simulink model "ROB_512_HW6_Hybrid"  (R2015a)
settings: Solver=ode23t  StartTime=0.0  StopTime=1.5  MaxStep=0.001  RelTol=1e-3
InitFcn:
  | Ka = 2;
  | Kb = 50;
libraries: fl_lib x17, nesl_utility x8, sh_lib x6, vrlib x3, simulink x2
Description:
  | Closed-Loop Electrohydraulic Actuator with Proportional Valve
  | 
  | This example shows an actuator that consists of a proportional 4-way directional valve
  | driving a double-acting hydraulic cylinder. The cylinder drives a load consisting of a mass,
  | viscous and Coulomb friction, constant force, and a spring. The actuator is powered
  | by a variable-displacement, pressure-compensated pump, driven by a constant velocity
  | motor. Pipelines between the valve, cylinder, pump, and the tank are simulated
  | with the Hydraulic Pipeline blocks.
  | 
  | 
  | Copyright 2008-2015 The MathWorks, Inc.
settings Model: ExtModeAutoUpdateStatusClock=off  Creator=MathWorks  LastModifiedBy=Ramsey
settings DataIOCC: SignalLoggingSaveFormat=ModelDataLogs
settings OptimizationCC: ExpressionDepthLimit=2147483647  InitFltsAndDblsToZero=on
settings DebuggingCC: SaveWithParameterizedLinksMsg=none  UnderspecifiedInitializationDetection=Classic  MergeDetectMultiDrivingBlocksExec=none  SignalResolutionControl=TryResolveAllWithWarning  SolverPrmCheckMsg=warning  MultiTaskDSMMsg=warning  FcnCallInpInsideContextMsg=UseLocalSettings  StateNameClashWarn=warning
settings GRTTargetCC: TargetFcnLib=ansi_tfl_tmw.mat  CombineOutputUpdateFcns=off  GRTInterface=on

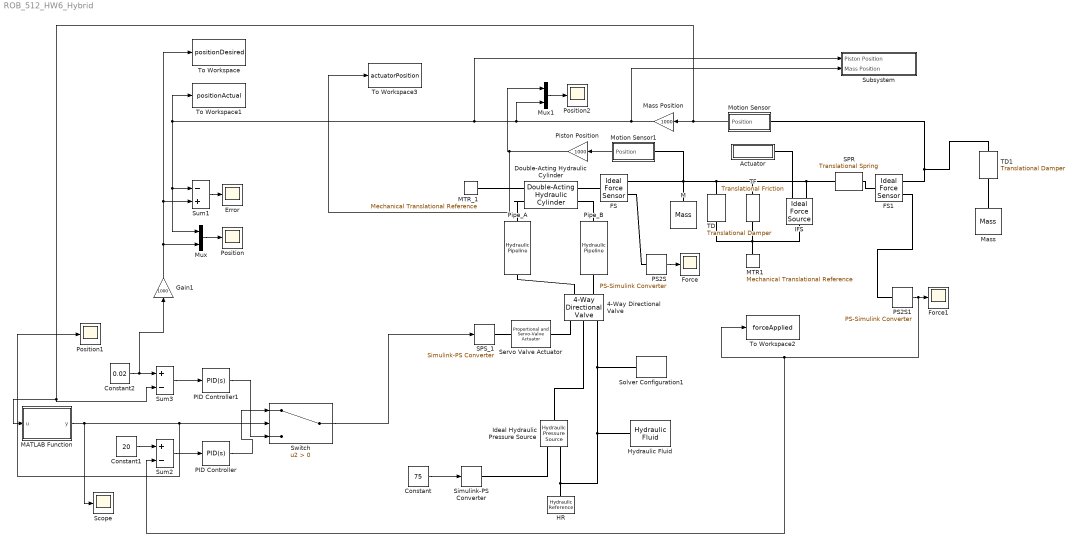
== system ROB_512_HW6_Hybrid ==
  4-Way Directional Valve : sh_lib/Valves/Directional Valves/4-Way Directional Valve  Tag=Factory Generic  mdl_type=1  area_max=0.00015 m^2  opening_max=0.01 m  opening_tab=[-0.002 0 0.005 0.015] m  area_tab=[1e-12 4e-12 1e-05 1.02e-05] m^2  pressure_tab=[-5000000 -2000000 2000000 5000000] Pa  flow_rate_tab=[-1e-12 -6e-14 6000000000000 100000000000;-8e-08 -4e-08 4000000 8000000;-0.0025 -0.00103 0.001 0.0024;-0.00258 -0.001032 0.00106 0.00247] m^3/s  interp_method=1  extrap_method=1  C_d=0.7  x_0_P_A=1e-05 m  x_0_P_B=1e-05 m  x_0_A_T=1e-05 m  x_0_B_T=1e-05 m  Re_cr=12  A_leak=1e-12 m^2
  Actuator : Subsystem
  Constant : Constant  Value=75
  Constant1 : Constant  Value=20
  Constant2 : Constant  Value=0.02
  Double-Acting Hydraulic Cylinder : sh_lib/Hydraulic Cylinders/Double-Acting Hydraulic Cylinder  Tag=Factory Generic  area_A=0.004 m^2  area_B=0.002 m^2  stroke=0.2 m  init_pos=0.1 m  dead_vol_A=0.001 m^3  dead_vol_B=0.001 m^3  init_pressure_A=0 Pa  init_pressure_B=0 Pa  k_sh=1.4  stiff=1e+12 N/m  D=150 N/(m/s)  or=1  or_sign=1
  Error : Scope
      settings: TimeRange=10  YMin=-0.01  YMax=0.02  MaxDataPoints=500000
  FS : fl_lib/Mechanical/Mechanical Sensors/Ideal Force Sensor  Tag=Factory Generic
  FS1 : fl_lib/Mechanical/Mechanical Sensors/Ideal Force Sensor  Tag=Factory Generic
  Force : Scope
      settings: TimeRange=3  YMin=-17500  YMax=27500  MaxDataPoints=500000
  Force1 : Scope
      settings: TimeRange=1.5  YMin=0  YMax=100  SaveName=ScopeData3  MaxDataPoints=500000
  Gain1 : Gain  Gain=1000
  HR : fl_lib/Hydraulic/Hydraulic Elements/Hydraulic Reference  Tag=Factory Generic
  Hydraulic Fluid : sh_lib/Hydraulic Utilities/Hydraulic Fluid  Tag=Factory Generic  DataSource=1  SelFluid=7  SysTemp=60 c  TrapAir=0.005  ViscDerFactor=1  range_error=2
  IFS : fl_lib/Mechanical/Mechanical Sources/Ideal Force Source  Tag=Factory Generic
  Ideal Hydraulic Pressure Source : fl_lib/Hydraulic/Hydraulic Sources/Hydraulic Pressure Source  Tag=Factory Generic
  M : fl_lib/Mechanical/Translational Elements/Mass  Tag=Factory Generic  mass=10 kg  v_specify=on  v_priority=High  v=0 m/s  f_specify=off  f_priority=High  f=0 N
  MATLAB Function : MATLAB Function  TreatAsAtomicUnit=on
  MTR1 : fl_lib/Mechanical/Translational Elements/Mechanical Translational Reference  Tag=Factory Generic
  MTR_1 : fl_lib/Mechanical/Translational Elements/Mechanical Translational Reference  Tag=Factory Generic
  Mass : fl_lib/Mechanical/Translational Elements/Mass  mass=5000 kg  v_specify=off  v_priority=High  v=0 m/s  f_specify=off  f_priority=High  f=0 N
  Mass Position : Gain  Gain=1000
  Motion Sensor : Subsystem
  Motion Sensor1 : Subsystem
  Mux : Mux  Inputs=2
  Mux1 : Mux  Inputs=2
  PID Controller : simulink/Continuous/PID Controller  Controller=PID  TimeDomain=Continuous-time  SampleTime=-1  IntegratorMethod=Forward Euler  FilterMethod=Forward Euler  Form=Parallel  UseFilter=on  ControllerParametersSource=internal  P=0.00035  I=0.00005  D=0  N=100  InitialConditionSource=internal  InitialConditionForIntegrator=0  InitialConditionForFilter=0  ExternalReset=none  LimitOutput=off  UpperSaturationLimit=inf  LowerSaturationLimit=-inf  LinearizeAsGain=on  AntiWindupMode=none  Kb=1  TrackingMode=off  Kt=1  PParamMin=[]  PParamMax=[]  IParamMin=[]  IParamMax=[]  DParamMin=[]  DParamMax=[]  NParamMin=[]  NParamMax=[]  KbParamMin=[]  KbParamMax=[]  KtParamMin=[]  KtParamMax=[]  POutMin=[]  POutMax=[]  IOutMin=[]  IOutMax=[]  DOutMin=[]  DOutMax=[]  NOutMin=[]  NOutMax=[]  KbOutMin=[]  KbOutMax=[]  KtOutMin=[]  KtOutMax=[]  IntegratorOutMin=[]  IntegratorOutMax=[]  FilterOutMin=[]  FilterOutMax=[]  SumOutMin=[]  SumOutMax=[]  SumI1OutMin=[]  SumI1OutMax=[]  SumI2OutMin=[]  SumI2OutMax=[]  SumI3OutMin=[]  SumI3OutMax=[]  SumDOutMin=[]  SumDOutMax=[]  SaturationOutMin=[]  SaturationOutMax=[]  IntegratorContinuousStateAttributes=''  IntegratorStateMustResolveToSignalObject=off  IntegratorRTWStateStorageClass=Auto  FilterContinuousStateAttributes=''  FilterStateMustResolveToSignalObject=off  FilterRTWStateStorageClass=Auto  DifferentiatorICPrevScaledInput=0  DifferentiatorOutMin=[]  DifferentiatorOutMax=[]
  PID Controller1 : simulink/Continuous/PID Controller  Controller=PID  TimeDomain=Continuous-time  SampleTime=-1  IntegratorMethod=Forward Euler  FilterMethod=Forward Euler  Form=Parallel  UseFilter=on  ControllerParametersSource=internal  P=5  I=0.1  D=0.2  N=100  InitialConditionSource=internal  InitialConditionForIntegrator=0  InitialConditionForFilter=0  ExternalReset=none  LimitOutput=off  UpperSaturationLimit=inf  LowerSaturationLimit=-inf  LinearizeAsGain=on  AntiWindupMode=none  Kb=1  TrackingMode=off  Kt=1  PParamMin=[]  PParamMax=[]  IParamMin=[]  IParamMax=[]  DParamMin=[]  DParamMax=[]  NParamMin=[]  NParamMax=[]  KbParamMin=[]  KbParamMax=[]  KtParamMin=[]  KtParamMax=[]  POutMin=[]  POutMax=[]  IOutMin=[]  IOutMax=[]  DOutMin=[]  DOutMax=[]  NOutMin=[]  NOutMax=[]  KbOutMin=[]  KbOutMax=[]  KtOutMin=[]  KtOutMax=[]  IntegratorOutMin=[]  IntegratorOutMax=[]  FilterOutMin=[]  FilterOutMax=[]  SumOutMin=[]  SumOutMax=[]  SumI1OutMin=[]  SumI1OutMax=[]  SumI2OutMin=[]  SumI2OutMax=[]  SumI3OutMin=[]  SumI3OutMax=[]  SumDOutMin=[]  SumDOutMax=[]  SaturationOutMin=[]  SaturationOutMax=[]  IntegratorContinuousStateAttributes=''  IntegratorStateMustResolveToSignalObject=off  IntegratorRTWStateStorageClass=Auto  FilterContinuousStateAttributes=''  FilterStateMustResolveToSignalObject=off  FilterRTWStateStorageClass=Auto  DifferentiatorICPrevScaledInput=0  DifferentiatorOutMin=[]  DifferentiatorOutMax=[]
  PS2S : nesl_utility/PS-Simulink Converter  PhysicalDomain=network_engine_domain  SubClassName=ps_output  LeftPortType=input  RightPortType=output  PseudoPeriodic=off  Frequencies=[]  Unit=1  AffineConversion=off
  PS2S1 : nesl_utility/PS-Simulink Converter  PhysicalDomain=network_engine_domain  SubClassName=ps_output  LeftPortType=input  RightPortType=output  PseudoPeriodic=off  Frequencies=[]  Unit=1  AffineConversion=off
  Pipe_A : sh_lib/Pipelines/Hydraulic Pipeline  Tag=Factory Generic  cs_type=1  d_in=0.02 m  area=0.0001 m^2  D_h=0.0112 m  s_factor=64  length=3 m  length_ad=2 m  roughness=1.5e-05 m  Re_lam=2000  Re_turb=4000  wall_type=1  pr_r_coef=2e-10 m/Pa  time_const=0.008 s  k_sh=1.4  initial_pressure=0 Pa
  Pipe_B : sh_lib/Pipelines/Hydraulic Pipeline  Tag=Factory Generic  cs_type=1  d_in=0.02 m  area=0.0001 m^2  D_h=0.0112 m  s_factor=64  length=3 m  length_ad=2 m  roughness=1.5e-05 m  Re_lam=2000  Re_turb=4000  wall_type=1  pr_r_coef=2e-10 m/Pa  time_const=0.008 s  k_sh=1.4  initial_pressure=0 Pa
  Piston Position : Gain  Gain=1000
  Position : Scope
      settings: TimeRange=1.5  YMin=2.5  YMax=20  SaveName=ScopeData2  MaxDataPoints=500000
  Position1 : Scope
      settings: TimeRange=3  YMin=1  YMax=1  SaveName=ScopeData5  MaxDataPoints=500000
  Position2 : Scope
      settings: ShowLegends=on  TimeRange=3  YMin=-10  YMax=150  SaveName=ScopeData6  MaxDataPoints=500000
  SPR : fl_lib/Mechanical/Translational Elements/Translational Spring  Tag=Factory Generic  spr_rate=1000 N/m  v_specify=off  v_priority=High  v=0 m/s  f_specify=off  f_priority=High  f=0 N  x_specify=on  x_priority=High  x=0 m
  SPS_1 : nesl_utility/Simulink-PS Converter  PhysicalDomain=network_engine_domain  SubClassName=ps_input  LeftPortType=input  RightPortType=output  PseudoPeriodic=off  Frequencies=[]  NoiseDistribution=none  NoiseParameters=[]  Unit=1  AffineConversion=off  InputFiltering=off  SimscapeFilterOrder=1  InputFilterTimeConstant=.001  UdotUserProvided=0
  Scope : Scope
      settings: SaveName=ScopeData4
  Servo Valve Actuator : sh_lib/Valves/Valve Actuators/Proportional and Servo-Valve Actuator  Tag=Factory Generic  gain=250  time_constant=0.002 s  saturation=0.3
  Simulink-PS Converter : nesl_utility/Simulink-PS Converter  PhysicalDomain=network_engine_domain  SubClassName=ps_input  LeftPortType=input  RightPortType=output  PseudoPeriodic=off  Frequencies=[]  NoiseDistribution=none  NoiseParameters=[]  Unit=bar  AffineConversion=off  InputFiltering=off  SimscapeFilterOrder=1  InputFilterTimeConstant=.001  UdotUserProvided=0
  Solver Configuration1 : nesl_utility/Solver Configuration  PhysicalDomain=network_engine_domain  SubClassName=solver  LeftPortType=input  RightPortType=generic  Accelerate=off  Tones=[]  Harmonics=[]  SimulateNoise=off  Profile=off  UseLocalSampling=off  EnableSwitchedLinearOptims=on  FrequencyDomain=off  UseCCode=off  RelTol=0.001  AbsTol=1e-06  MinStep=1e-09  ToWorkspace=off  RevertToSquareIcSolve=off  NumHomotopyIterations=100  DoDC=off  ResidualTolerance=1e-9  UseLocalSolver=off  LocalSolverChoice=NE_BACKWARD_EULER_ADVANCER  LocalSolverSampleTime=.001  DoFixedCost=off  MaxNonlinIter=3  MaxModeIter=2  LinearAlgebra=Sparse  DelaysMemoryBudget=1024  AutomaticFiltering=on  FilteringTimeConstant=0.001
  Subsystem : Subsystem
  Sum1 : Sum  Inputs=-+
  Sum2 : Sum  Inputs=+-
  Sum3 : Sum  Inputs=+-
  Switch : Switch  Criteria=u2 > Threshold  RndMeth=Round  ZeroCross=off
  TD : fl_lib/Mechanical/Translational Elements/Translational Damper  Tag=Factory Generic  D=2 N/(m/s)  v_specify=off  v_priority=High  v=0 m/s  f_specify=off  f_priority=High  f=0 N
  TD1 : fl_lib/Mechanical/Translational Elements/Translational Damper  Tag=Factory Generic  D=500 N/(m/s)  v_specify=off  v_priority=High  v=0 m/s  f_specify=off  f_priority=High  f=0 N
  TF : fl_lib/Mechanical/Translational Elements/Translational Friction  Tag=Factory Generic  brkwy_frc=500 N  Col_frc=500 N  visc_coef=0.01 N/(m/s)  trans_coef=10 s/m  vel_thr=0.0001 m/s  v_specify=off  v_priority=High  v=0 m/s  f_specify=off  f_priority=High  f=0 N
  To Workspace : ToWorkspace  VariableName=positionDesired  SaveFormat=Timeseries  SampleTime=-1
  To Workspace1 : ToWorkspace  VariableName=positionActual  SaveFormat=Timeseries  SampleTime=-1
  To Workspace2 : ToWorkspace  VariableName=forceApplied  SaveFormat=Timeseries  SampleTime=-1
  To Workspace3 : ToWorkspace  VariableName=actuatorPosition  SaveFormat=Timeseries  SampleTime=-1
  wires:
  PS2S/1 -> Force/1
  Constant1/1 -> Sum2/1
  Mux/1 -> Position/1
  Sum1/1 -> Error/1
  Constant/1 -> Simulink-PS Converter/1
  Gain1/1 -> To Workspace/1, Sum1/2, Mux/2
  PS2S1/1 -> To Workspace2/1, Sum2/2, Force1/1
  Sum2/1 -> PID Controller/1
  Constant2/1 -> Gain1/1, Sum3/1
  Sum3/1 -> PID Controller1/1
  Motion Sensor/1(Position) -> Mass Position/1, MATLAB Function/1(u), Sum3/2
  PID Controller/1 -> Switch/1
  PID Controller1/1 -> Switch/3
  Switch/1 -> SPS_1/1
  MATLAB Function/1(y) -> Scope/1, Position1/1, Switch/2
  Mux1/1 -> Position2/1
  Motion Sensor1/1(Position) -> Piston Position/1
  Piston Position/1 -> To Workspace3/1, Mux1/1
  Mass Position/1 -> Subsystem/2(Mass Position), Mux1/2, Subsystem/1(Piston Position), Mux/1, Sum1/1, To Workspace1/1
  connections:
  MTR_1/LConn1 -- Double-Acting Hydraulic Cylinder/LConn1
  FS/LConn1 -- Double-Acting Hydraulic Cylinder/RConn1
  FS/RConn2 -- PS2S/LConn1
  Ideal Hydraulic Pressure Source/RConn2 -- Hydraulic Fluid/RConn1 -- Solver Configuration1/RConn1 -- 4-Way Directional Valve/RConn3 -- HR/LConn1
  4-Way Directional Valve/RConn1 -- Servo Valve Actuator/RConn1
  SPS_1/RConn1 -- Servo Valve Actuator/LConn1
  Ideal Hydraulic Pressure Source/LConn1 -- 4-Way Directional Valve/RConn2
  SPR/LConn1 -- IFS/RConn2 -- TD/LConn1 -- Motion Sensor1/LConn1 -- M/LConn1 -- FS/RConn1 -- TF/LConn1
  Actuator/RConn1 -- IFS/RConn1
  TD/RConn1 -- TF/RConn1 -- IFS/LConn1 -- MTR1/LConn1
  Simulink-PS Converter/RConn1 -- Ideal Hydraulic Pressure Source/RConn1
  Double-Acting Hydraulic Cylinder/LConn2 -- Pipe_A/RConn1
  4-Way Directional Valve/LConn1 -- Pipe_A/LConn1
  Double-Acting Hydraulic Cylinder/RConn2 -- Pipe_B/LConn1
  4-Way Directional Valve/LConn2 -- Pipe_B/RConn1
  FS1/LConn1 -- SPR/RConn1
  Motion Sensor/LConn1 -- TD1/LConn1 -- FS1/RConn1
  FS1/RConn2 -- PS2S1/LConn1
  Mass/LConn1 -- TD1/RConn1

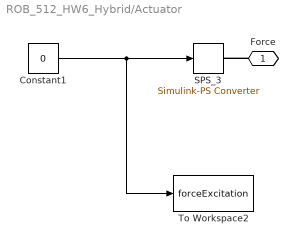
== system ROB_512_HW6_Hybrid/Actuator ==
  Constant1 : Constant  Value=0
  SPS_3 : nesl_utility/Simulink-PS Converter  PhysicalDomain=network_engine_domain  SubClassName=ps_input  LeftPortType=input  RightPortType=output  PseudoPeriodic=off  Frequencies=[]  NoiseDistribution=none  NoiseParameters=[]  Unit=1  AffineConversion=off  InputFiltering=off  SimscapeFilterOrder=1  InputFilterTimeConstant=.001  UdotUserProvided=0
  To Workspace2 : ToWorkspace  VariableName=forceExcitation  SaveFormat=Timeseries  SampleTime=-1
  Force : PMIOPort  Port=1  Side=Right
  wires:
  Constant1/1 -> To Workspace2/1, SPS_3/1
  connections:
  Force/RConn1 -- SPS_3/RConn1

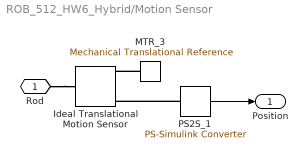
== system ROB_512_HW6_Hybrid/Motion Sensor ==
  Ideal Translational Motion Sensor : fl_lib/Mechanical/Mechanical Sensors/Ideal Translational Motion Sensor  Tag=Factory Generic  offset=0 m
  MTR_3 : fl_lib/Mechanical/Translational Elements/Mechanical Translational Reference  Tag=Factory Generic
  PS2S_1 : nesl_utility/PS-Simulink Converter  PhysicalDomain=network_engine_domain  SubClassName=ps_output  LeftPortType=input  RightPortType=output  PseudoPeriodic=off  Frequencies=[]  Unit=1  AffineConversion=off
  Rod : PMIOPort  Port=1  Side=Left
  Position : Outport
  wires:
  PS2S_1/1 -> Position/1
  connections:
  Rod/RConn1 -- Ideal Translational Motion Sensor/LConn1
  PS2S_1/LConn1 -- Ideal Translational Motion Sensor/RConn3
  MTR_3/LConn1 -- Ideal Translational Motion Sensor/RConn1

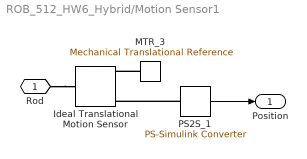
== system ROB_512_HW6_Hybrid/Motion Sensor1 ==
  Ideal Translational Motion Sensor : fl_lib/Mechanical/Mechanical Sensors/Ideal Translational Motion Sensor  Tag=Factory Generic  offset=0 m
  MTR_3 : fl_lib/Mechanical/Translational Elements/Mechanical Translational Reference  Tag=Factory Generic
  PS2S_1 : nesl_utility/PS-Simulink Converter  PhysicalDomain=network_engine_domain  SubClassName=ps_output  LeftPortType=input  RightPortType=output  PseudoPeriodic=off  Frequencies=[]  Unit=1  AffineConversion=off
  Rod : PMIOPort  Port=1  Side=Left
  Position : Outport
  wires:
  PS2S_1/1 -> Position/1
  connections:
  Rod/RConn1 -- Ideal Translational Motion Sensor/LConn1
  PS2S_1/LConn1 -- Ideal Translational Motion Sensor/RConn3
  MTR_3/LConn1 -- Ideal Translational Motion Sensor/RConn1

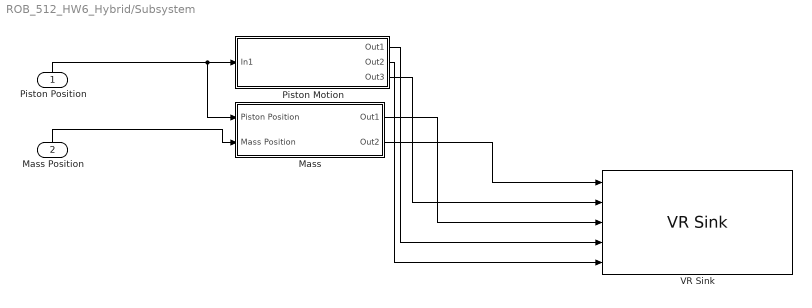
== system ROB_512_HW6_Hybrid/Subsystem ==
  Piston Position : Inport
  Mass Position : Inport  Port=2
  "Mass " : Subsystem
  Piston Motion : Subsystem
  VR Sink : vrlib/VR Sink  InstantiateOnLoad=on  SampleTime=0.001  ViewEnable=on  RemoteChange=off  RemoteView=off  FieldsWritten=Spring.scale.3.1.1.double#Spring.translation.3.1.1.double#Box.translation.3.1.1.double#Puck.translation.3.1.1.double#Piston.translation.3.1.1.double  WorldFileName=Force_Control_Simulation.WRL  AutoView=off  VideoDimensions=[]  AllowVariableSize=off
  wires:
  Piston Motion/2(Out2) -> VR Sink/5
  "Mass "/2(Out2) -> VR Sink/1
  "Mass "/1(Out1) -> VR Sink/3
  Piston Motion/1(Out1) -> VR Sink/4
  Piston Motion/3(Out3) -> VR Sink/2
  Piston Position/1 -> "Mass "/1(Piston Position), Piston Motion/1(In1)
  Mass Position/1 -> "Mass "/2(Mass Position)

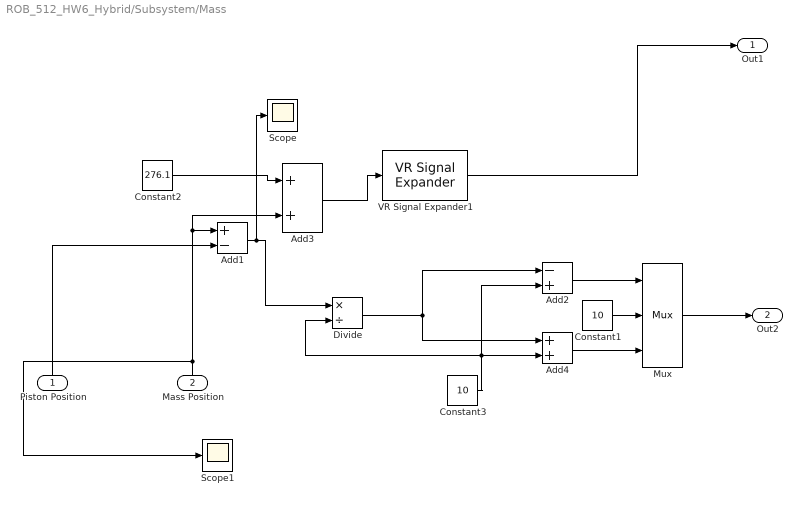
== system ROB_512_HW6_Hybrid/Subsystem/Mass  ==
  Piston Position : Inport
  Mass Position : Inport  Port=2
  Add1 : Sum  Inputs=+-
  Add2 : Sum  Inputs=-+
  Add3 : Sum
  Add4 : Sum
  Constant1 : Constant  Value=10
  Constant2 : Constant  Value=276.1
  Constant3 : Constant  Value=10
  Divide : Product  Inputs=*/
  Mux : Mux  Inputs=3
  Scope : Scope
      settings: YMin=-44.2  YMax=-41.8  SaveName=ScopeData4
  Scope1 : Scope
      settings: YMin=-44.2  YMax=-41.8  SaveName=ScopeData6
  VR Signal Expander1 : vrlib/VR Signal Expander  outwidth=3  outidx=[1]
  Out1 : Outport
  Out2 : Outport  Port=2
  wires:
  Constant2/1 -> Add3/1
  VR Signal Expander1/1 -> Out1/1
  Piston Position/1 -> Add1/2
  Mass Position/1 -> Add1/1, Add3/2, Scope1/1
  Add3/1 -> VR Signal Expander1/1
  Constant1/1 -> Mux/2
  Mux/1 -> Out2/1
  Add1/1 -> Scope/1, Divide/1
  Add4/1 -> Mux/3
  Add2/1 -> Mux/1
  Constant3/1 -> Divide/2, Add2/2, Add4/2
  Divide/1 -> Add2/1, Add4/1

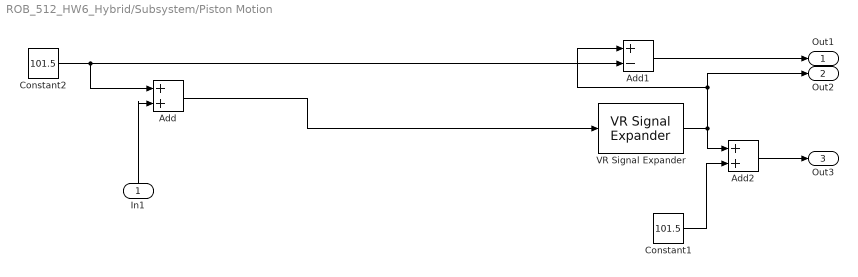
== system ROB_512_HW6_Hybrid/Subsystem/Piston Motion ==
  In1 : Inport
  Add : Sum
  Add1 : Sum  Inputs=+-
  Add2 : Sum
  Constant1 : Constant  Value=101.5
  Constant2 : Constant  Value=101.5
  VR Signal Expander : vrlib/VR Signal Expander  outwidth=3  outidx=[1]
  Out1 : Outport
  Out2 : Outport  Port=2
  Out3 : Outport  Port=3
  wires:
  Constant2/1 -> Add/1, Add1/2
  Add/1 -> VR Signal Expander/1
  VR Signal Expander/1 -> Add2/1, Out2/1, Add1/1
  Add1/1 -> Out1/1
  In1/1 -> Add/2
  Add2/1 -> Out3/1
  Constant1/1 -> Add2/2

== matlab function ROB_512_HW6_Hybrid/MATLAB Function ==
  data: u input; y output
function y = fcn(u)

if u > 0.02
    
    
    y = 1;
else
    y = 0;
end
